simulink model "OutputMVA"  (Simulink 8.7)
settings: Solver=ode45  StartTime=0.0  StopTime=10.0  RelTol=1e-3
undefined symbols (not defined in the file or in its folder): sMP
(part 2 of 3)

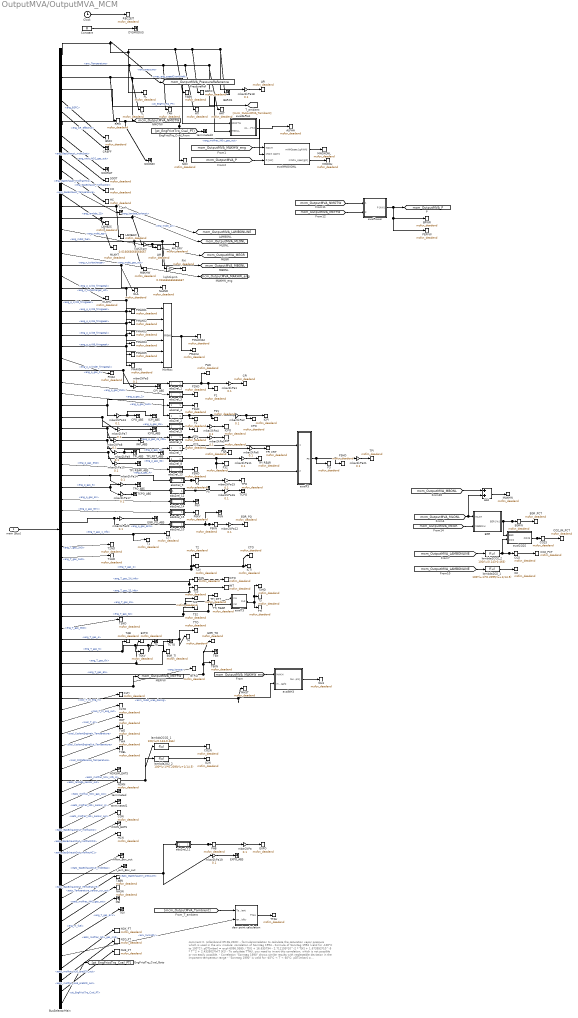
== system OutputMVA/OutputMVA_MCM ==
  note: comment C. Hillenbrand 09.06.2020:
      |
      | - formula/correlation to calculate the saturation vapor pressure which is used in the env module: correlation of Sonntag 1994
      | - Formula of Sonntag 1994 (valid for -100°C to 100°C): pDT[mbar] = exp(-6096.9385 / T[K] + 16.635794 - 2.711193*10^-2 * T[K] + 1.673952*10^-5 * T^2 + 2.433502*ln(T [K])
      | - To calculate TTAU, you need to invert this correlation, which is not possible or not easily possible.
      |
      | - Correlation "Sonntag 1990" shows similar results with neglectable deviation in the important temperatur range
      | - "Sonntag 1990" is valid for -45°C < T < 60°C:  pDT[mbar] = 6.112*exp((17.62*T)/(243.12+T))
      | - TTAU calculation:
      |                  h = pDT(TTAU) / pDT(T)
      |                  TTAU [°C] = 243.12 * ((17.62*T)/(243.12 + T) +ln(h))/((17.62*243.12)/(243.12 + T) -ln(h))   T=ambient temperatur    h=humidity
      |              (source: Beat P. Kneubuehl, "Ballistik: Theorie und Praxis" --> Kapitel 5.2.2 (Seite 155)
      |                           https://books.google.de/books?id=MtSBDwAAQBAJ&pg=PA155&lpg=PA155&dq=magnus+formel+s%C3%A4ttigungsdampfdruck+ballistik&source=bl&ots=gXIhdY-Apv&sig=ACfU3U0MpvOVRWRlQYtERQ3iZreJqlAHjg&hl=de&sa=X&ved=2ahUKEwic3uGe9fTpAhVzwcQBHcHJBsQQ6AEwAXoECAoQAQ#v=onepage&q=magnus%20formel%20s%C3%A4ttigungsdampfdruck%20ballistik&f=false
      |                      or: https://de.wikipedia.org/wiki/Sättigungsdampfdruck    --> Magnus-Formel)
      |
      |
      | --> The two correlations ("Sonntag 1994" and "Sonntag 1990" show results with negectable deviations in the important temperature range compared to MVAPC correlation.
      | --> Correlation "Sonntag 1994" will still be implemented in the environment modul.
      | --> For TTAU calculation "Sonntag 1990" will be used, due to the possible inversion the correlation.
  main [Bus] : Inport
  ALPHA : M-S-Function  Tag=VTOS_ALPHA  FunctionName=msfcn_deadend  mask(S-function: msfcn_deadend){}
      mask help: This is a level-2 M file S-function for communication with a VITOS (Virtual Testbench Operating System) display GUI element.
      mask Help: This is a level-2 M file S-function for communication with a VITOS (Virtual Testbench Operating System) display GUI element.
      mask Display: disp(['V'])
  AM : M-S-Function  Tag=VTOS_AM  FunctionName=msfcn_deadend  mask(S-function: msfcn_deadend){}
      mask help: This is a level-2 M file S-function for communication with a VITOS (Virtual Testbench Operating System) display GUI element.
      mask Help: This is a level-2 M file S-function for communication with a VITOS (Virtual Testbench Operating System) display GUI element.
      mask Display: disp(['V'])
  AMT : M-S-Function  Tag=VTOS_AMT  FunctionName=msfcn_deadend  mask(S-function: msfcn_deadend){}
      mask help: This is a level-2 M file S-function for communication with a VITOS (Virtual Testbench Operating System) display GUI element.
      mask Help: This is a level-2 M file S-function for communication with a VITOS (Virtual Testbench Operating System) display GUI element.
      mask Display: disp(['V'])
  AM_DRY : M-S-Function  Tag=VTOS_AM_DRY  FunctionName=msfcn_deadend  mask(S-function: msfcn_deadend){}
      mask help: This is a level-2 M file S-function for communication with a VITOS (Virtual Testbench Operating System) display GUI element.
      mask Help: This is a level-2 M file S-function for communication with a VITOS (Virtual Testbench Operating System) display GUI element.
      mask Display: disp(['V'])
  API : M-S-Function  Tag=VTOS_API  FunctionName=msfcn_deadend  mask(S-function: msfcn_deadend){}
      mask help: This is a level-2 M file S-function for communication with a VITOS (Virtual Testbench Operating System) display GUI element.
      mask Help: This is a level-2 M file S-function for communication with a VITOS (Virtual Testbench Operating System) display GUI element.
      mask Display: disp(['V'])
  ATI : M-S-Function  Tag=VTOS_ATI  FunctionName=msfcn_deadend  mask(S-function: msfcn_deadend){}
      mask help: This is a level-2 M file S-function for communication with a VITOS (Virtual Testbench Operating System) display GUI element.
      mask Help: This is a level-2 M file S-function for communication with a VITOS (Virtual Testbench Operating System) display GUI element.
      mask Display: disp(['V'])
  Add : Sum
  BARO : M-S-Function  Tag=VTOS_BARO  FunctionName=msfcn_deadend  mask(S-function: msfcn_deadend){}
      mask help: This is a level-2 M file S-function for communication with a VITOS (Virtual Testbench Operating System) display GUI element.
      mask Help: This is a level-2 M file S-function for communication with a VITOS (Virtual Testbench Operating System) display GUI element.
      mask Display: disp(['V'])
  BARO1 : Terminator
  BPWR : M-S-Function  Tag=VTOS_BPWR  FunctionName=msfcn_deadend  mask(S-function: msfcn_deadend){}
      mask help: This is a level-2 M file S-function for communication with a VITOS (Virtual Testbench Operating System) display GUI element.
      mask Help: This is a level-2 M file S-function for communication with a VITOS (Virtual Testbench Operating System) display GUI element.
      mask Display: disp(['V'])
  BSFC : M-S-Function  Tag=VTOS_BSFC  FunctionName=msfcn_deadend  mask(S-function: msfcn_deadend){}
      mask help: This is a level-2 M file S-function for communication with a VITOS (Virtual Testbench Operating System) display GUI element.
      mask Help: This is a level-2 M file S-function for communication with a VITOS (Virtual Testbench Operating System) display GUI element.
      mask Display: disp(['V'])
  BTRQ : M-S-Function  Tag=VTOS_BTRQ  FunctionName=msfcn_deadend  mask(S-function: msfcn_deadend){}
      mask help: This is a level-2 M file S-function for communication with a VITOS (Virtual Testbench Operating System) display GUI element.
      mask Help: This is a level-2 M file S-function for communication with a VITOS (Virtual Testbench Operating System) display GUI element.
      mask Display: disp(['V'])
  BusSelectorMain : BusSelector  OutputSignals=boundary [Bus].env_pressure,boundary [Bus].env_Temperature,sensor [Bus].mec_eng_speedCrankshaft,control [Bus].pt_EngTrq_Rq_PT,info [Bus].eng_BSFC,info [Bus].eng_CR_effective,sensor [Bus].eng_molfrac_NOx_gas_out,info [Bus].eng_ratio_NO2_gas_out,physics [Bus].eng_GasExhaust_mdotSoot,physics [Bus].eng_GasExhaust_molfracCO,physics [Bus].eng_GasExhaust_molfracHC1,physics [Bus].eng_GasExhaust_Temperature,info [Bus].eng_lambda_2S,sensor [Bus].eng_lambda_exhaust,sensor [Bus].eng_mdot_air,sensor [Bus].eng_mdot_egr,info [Bus].eng_mdot_fuel,sensor [Bus].eng_mdot_gas_out,sensor [Bus].eng_n_turbocharger,sensor [Bus].eng_n_turbocharger_HP,info [Bus].eng_p_cyl01_firingpeak,info [Bus].eng_p_cyl02_firingpeak,info [Bus].eng_p_cyl03_firingpeak,info [Bus].eng_p_cyl04_firingpeak,info [Bus].eng_p_cyl05_firingpeak,info [Bus].eng_p_cyl06_firingpeak,info [Bus].eng_p_cylinder_firingpeak,info [Bus].eng_p_gas_1,info [Bus].eng_p_gas_2ND,info [Bus].eng_p_gas_1HD,info [Bus].eng_p_gas_2,sensor [Bus].eng_p_gas_2N,info [Bus].eng_p_gas_2S_info,sensor [Bus].eng_p_gas_31,info [Bus].eng_p_gas_32,info [Bus].eng_p_gas_3ND,sensor [Bus].eng_p_gas_4,info [Bus].eng_p_gas_5,info [Bus].eng_p_gas_6V,info [Bus].eng_p_gas_6KV,sensor [Bus].eng_p_gas_6KN,info [Bus].eng_T_gas_1_info,info [Bus].eng_T_gas_2ND,info [Bus].eng_T_gas_1HD,sensor [Bus].eng_T_gas_2,info [Bus].eng_T_gas_2N_info,info [Bus].eng_T_gas_2S_info,sensor [Bus].eng_T_gas_31,sensor [Bus].eng_T_gas_32,info [Bus].eng_T_gas_3ND,sensor [Bus].eng_T_gas_4,info [Bus].eng_T_gas_5,info [Bus].eng_T_gas_6V,sensor [Bus].eng_T_gas_6N,sensor [Bus].eng_torque,actuator [Bus].acm_mdot_urea_dosing,sensor [Bus].cool_T_ct_eng_in,sensor [Bus].cool_T_ct_eng_out,sensor [Bus].cool_T_oil,physics [Bus].cool_CoolantEngineIn_Temperature,physics [Bus].cool_CoolantEngineOut_Temperature,physics [Bus].cool_OilReference_Temperature,sensor [Bus].eats_lambda_sensor_out,info [Bus].eats_molfrac_NOx_info_in,info [Bus].eats_molfrac_NOx_gas_out,sensor [Bus].eats_molfrac_NOx_sensor_in,sensor [Bus].eats_molfrac_NOx_sensor_out,physics [Bus].eats_GasExhaustOut_molfracCO,physics [Bus].eats_GasExhaustOut_molfracCO2,physics [Bus].eats_GasExhaustOut_molfracHC1,physics [Bus].eats_GasExhaustIn_pressure,physics [Bus].eats_GasExhaustOut_mdotGas,physics [Bus].eats_GasExhaustOut_Temperature,sensor [Bus].eats_Temperature_sensor_scr_out,info [Bus].eats_molfrac_NH3_gas_out,info [Bus].eng_m_fuel,info [Bus].eng_T_gas_6VV,boundary [Bus].env_humidity,info [Bus].eats_molfrac_NOx_gas_mid,info [Bus].eats_molfrac_N2O_preSCR_out,info [Bus].eats_molfrac_NH3_preSCR_out, control [Bus].pt_EngFrictTrq_Cval_PT
  CLTI : M-S-Function  Tag=VTOS_CLTI  FunctionName=msfcn_deadend  mask(S-function: msfcn_deadend){}
      mask help: This is a level-2 M file S-function for communication with a VITOS (Virtual Testbench Operating System) display GUI element.
      mask Help: This is a level-2 M file S-function for communication with a VITOS (Virtual Testbench Operating System) display GUI element.
      mask Display: disp(['V'])
  CLTO : M-S-Function  Tag=VTOS_CLTO  FunctionName=msfcn_deadend  mask(S-function: msfcn_deadend){}
      mask help: This is a level-2 M file S-function for communication with a VITOS (Virtual Testbench Operating System) display GUI element.
      mask Help: This is a level-2 M file S-function for communication with a VITOS (Virtual Testbench Operating System) display GUI element.
      mask Display: disp(['V'])
  CO : M-S-Function  Tag=VTOS_CO  FunctionName=msfcn_deadend  mask(S-function: msfcn_deadend){}
      mask help: This is a level-2 M file S-function for communication with a VITOS (Virtual Testbench Operating System) display GUI element.
      mask Help: This is a level-2 M file S-function for communication with a VITOS (Virtual Testbench Operating System) display GUI element.
      mask Display: disp(['V'])
  CO2 : M-S-Function  Tag=VTOS_CO2  FunctionName=msfcn_deadend  mask(S-function: msfcn_deadend){}
      mask help: This is a level-2 M file S-function for communication with a VITOS (Virtual Testbench Operating System) display GUI element.
      mask Help: This is a level-2 M file S-function for communication with a VITOS (Virtual Testbench Operating System) display GUI element.
      mask Display: disp(['V'])
  CO2N : M-S-Function  Tag=VTOS_CO2N  FunctionName=msfcn_deadend  mask(S-function: msfcn_deadend){}
      mask help: This is a level-2 M file S-function for communication with a VITOS (Virtual Testbench Operating System) display GUI element.
      mask Help: This is a level-2 M file S-function for communication with a VITOS (Virtual Testbench Operating System) display GUI element.
      mask Display: disp(['V'])
  CO2N_EATS : Terminator
  CO2S : M-S-Function  Tag=VTOS_CO2S  FunctionName=msfcn_deadend  mask(S-function: msfcn_deadend){}
      mask help: This is a level-2 M file S-function for communication with a VITOS (Virtual Testbench Operating System) display GUI element.
      mask Help: This is a level-2 M file S-function for communication with a VITOS (Virtual Testbench Operating System) display GUI element.
      mask Display: disp(['V'])
  CO2_IM_PCT : M-S-Function  Tag=VTOS_CO2_IM_PCT  FunctionName=msfcn_deadend  mask(S-function: msfcn_deadend){}
      mask help: This is a level-2 M file S-function for communication with a VITOS (Virtual Testbench Operating System) display GUI element.
      mask Help: This is a level-2 M file S-function for communication with a VITOS (Virtual Testbench Operating System) display GUI element.
      mask Display: disp(['V'])
  CO2_PCT : M-S-Function  Tag=VTOS_CO2_PCT  FunctionName=msfcn_deadend  mask(S-function: msfcn_deadend){}
      mask help: This is a level-2 M file S-function for communication with a VITOS (Virtual Testbench Operating System) display GUI element.
      mask Help: This is a level-2 M file S-function for communication with a VITOS (Virtual Testbench Operating System) display GUI element.
      mask Display: disp(['V'])
  CON : M-S-Function  Tag=VTOS_CON  FunctionName=msfcn_deadend  mask(S-function: msfcn_deadend){}
      mask help: This is a level-2 M file S-function for communication with a VITOS (Virtual Testbench Operating System) display GUI element.
      mask Help: This is a level-2 M file S-function for communication with a VITOS (Virtual Testbench Operating System) display GUI element.
      mask Display: disp(['V'])
  CPI : M-S-Function  Tag=VTOS_CPI  FunctionName=msfcn_deadend  mask(S-function: msfcn_deadend){}
      mask help: This is a level-2 M file S-function for communication with a VITOS (Virtual Testbench Operating System) display GUI element.
      mask Help: This is a level-2 M file S-function for communication with a VITOS (Virtual Testbench Operating System) display GUI element.
      mask Display: disp(['V'])
  CPI_ABS : Terminator
  CPO : M-S-Function  Tag=VTOS_CPO  FunctionName=msfcn_deadend  mask(S-function: msfcn_deadend){}
      mask help: This is a level-2 M file S-function for communication with a VITOS (Virtual Testbench Operating System) display GUI element.
      mask Help: This is a level-2 M file S-function for communication with a VITOS (Virtual Testbench Operating System) display GUI element.
      mask Display: disp(['V'])
  CPO_ABS : Terminator
  CREFF : Terminator
  CTI : M-S-Function  Tag=VTOS_CTI  FunctionName=msfcn_deadend  mask(S-function: msfcn_deadend){}
      mask help: This is a level-2 M file S-function for communication with a VITOS (Virtual Testbench Operating System) display GUI element.
      mask Help: This is a level-2 M file S-function for communication with a VITOS (Virtual Testbench Operating System) display GUI element.
      mask Display: disp(['V'])
  CTO : M-S-Function  Tag=VTOS_CTO  FunctionName=msfcn_deadend  mask(S-function: msfcn_deadend){}
      mask help: This is a level-2 M file S-function for communication with a VITOS (Virtual Testbench Operating System) display GUI element.
      mask Help: This is a level-2 M file S-function for communication with a VITOS (Virtual Testbench Operating System) display GUI element.
      mask Display: disp(['V'])
  Clock : Clock
  Constant : Constant  Value=8
  DYSMODUS : Terminator
  EGR : Subsystem
  EGRW : M-S-Function  Tag=VTOS_EGRW  FunctionName=msfcn_deadend  mask(S-function: msfcn_deadend){}
      mask help: This is a level-2 M file S-function for communication with a VITOS (Virtual Testbench Operating System) display GUI element.
      mask Help: This is a level-2 M file S-function for communication with a VITOS (Virtual Testbench Operating System) display GUI element.
      mask Display: disp(['V'])
  EGR_PCT : M-S-Function  Tag=VTOS_EGR_PCT  FunctionName=msfcn_deadend  mask(S-function: msfcn_deadend){}
      mask help: This is a level-2 M file S-function for communication with a VITOS (Virtual Testbench Operating System) display GUI element.
      mask Help: This is a level-2 M file S-function for communication with a VITOS (Virtual Testbench Operating System) display GUI element.
      mask Display: disp(['V'])
  EGR_PO : M-S-Function  Tag=VTOS_EGR_PO  FunctionName=msfcn_deadend  mask(S-function: msfcn_deadend){}
      mask help: This is a level-2 M file S-function for communication with a VITOS (Virtual Testbench Operating System) display GUI element.
      mask Help: This is a level-2 M file S-function for communication with a VITOS (Virtual Testbench Operating System) display GUI element.
      mask Display: disp(['V'])
  EGR_PO_ABS : Terminator
  EGR_TI : M-S-Function  Tag=VTOS_EGR_TI  FunctionName=msfcn_deadend  mask(S-function: msfcn_deadend){}
      mask help: This is a level-2 M file S-function for communication with a VITOS (Virtual Testbench Operating System) display GUI element.
      mask Help: This is a level-2 M file S-function for communication with a VITOS (Virtual Testbench Operating System) display GUI element.
      mask Display: disp(['V'])
  EGR_TO : M-S-Function  Tag=VTOS_EGR_TO  FunctionName=msfcn_deadend  mask(S-function: msfcn_deadend){}
      mask help: This is a level-2 M file S-function for communication with a VITOS (Virtual Testbench Operating System) display GUI element.
      mask Help: This is a level-2 M file S-function for communication with a VITOS (Virtual Testbench Operating System) display GUI element.
      mask Display: disp(['V'])
  EXPO : M-S-Function  Tag=VTOS_EXPO  FunctionName=msfcn_deadend  mask(S-function: msfcn_deadend){}
      mask help: This is a level-2 M file S-function for communication with a VITOS (Virtual Testbench Operating System) display GUI element.
      mask Help: This is a level-2 M file S-function for communication with a VITOS (Virtual Testbench Operating System) display GUI element.
      mask Display: disp(['V'])
  EXPO_ABS : Terminator
  EXTO : M-S-Function  Tag=VTOS_EXTO  FunctionName=msfcn_deadend  mask(S-function: msfcn_deadend){}
      mask help: This is a level-2 M file S-function for communication with a VITOS (Virtual Testbench Operating System) display GUI element.
      mask Help: This is a level-2 M file S-function for communication with a VITOS (Virtual Testbench Operating System) display GUI element.
      mask Display: disp(['V'])
  FM : M-S-Function  Tag=VTOS_FM  FunctionName=msfcn_deadend  mask(S-function: msfcn_deadend){}
      mask help: This is a level-2 M file S-function for communication with a VITOS (Virtual Testbench Operating System) display GUI element.
      mask Help: This is a level-2 M file S-function for communication with a VITOS (Virtual Testbench Operating System) display GUI element.
      mask Display: disp(['V'])
  GOT : M-S-Function  Tag=VTOS_GOT  FunctionName=msfcn_deadend  mask(S-function: msfcn_deadend){}
      mask help: This is a level-2 M file S-function for communication with a VITOS (Virtual Testbench Operating System) display GUI element.
      mask Help: This is a level-2 M file S-function for communication with a VITOS (Virtual Testbench Operating System) display GUI element.
      mask Display: disp(['V'])
  HC : M-S-Function  Tag=VTOS_HC  FunctionName=msfcn_deadend  mask(S-function: msfcn_deadend){}
      mask help: This is a level-2 M file S-function for communication with a VITOS (Virtual Testbench Operating System) display GUI element.
      mask Help: This is a level-2 M file S-function for communication with a VITOS (Virtual Testbench Operating System) display GUI element.
      mask Display: disp(['V'])
  HCN : M-S-Function  Tag=VTOS_HCN  FunctionName=msfcn_deadend  mask(S-function: msfcn_deadend){}
      mask help: This is a level-2 M file S-function for communication with a VITOS (Virtual Testbench Operating System) display GUI element.
      mask Help: This is a level-2 M file S-function for communication with a VITOS (Virtual Testbench Operating System) display GUI element.
      mask Display: disp(['V'])
  ICPI : M-S-Function  Tag=VTOS_ICPI  FunctionName=msfcn_deadend  mask(S-function: msfcn_deadend){}
      mask help: This is a level-2 M file S-function for communication with a VITOS (Virtual Testbench Operating System) display GUI element.
      mask Help: This is a level-2 M file S-function for communication with a VITOS (Virtual Testbench Operating System) display GUI element.
      mask Display: disp(['V'])
  ICPI_ABS : Terminator
  ICPO : M-S-Function  Tag=VTOS_ICPO  FunctionName=msfcn_deadend  mask(S-function: msfcn_deadend){}
      mask help: This is a level-2 M file S-function for communication with a VITOS (Virtual Testbench Operating System) display GUI element.
      mask Help: This is a level-2 M file S-function for communication with a VITOS (Virtual Testbench Operating System) display GUI element.
      mask Display: disp(['V'])
  ICPO_ABS : Terminator
  ICTI : M-S-Function  Tag=VTOS_ICTI  FunctionName=msfcn_deadend  mask(S-function: msfcn_deadend){}
      mask help: This is a level-2 M file S-function for communication with a VITOS (Virtual Testbench Operating System) display GUI element.
      mask Help: This is a level-2 M file S-function for communication with a VITOS (Virtual Testbench Operating System) display GUI element.
      mask Display: disp(['V'])
  ICTO : M-S-Function  Tag=VTOS_ICTO  FunctionName=msfcn_deadend  mask(S-function: msfcn_deadend){}
      mask help: This is a level-2 M file S-function for communication with a VITOS (Virtual Testbench Operating System) display GUI element.
      mask Help: This is a level-2 M file S-function for communication with a VITOS (Virtual Testbench Operating System) display GUI element.
      mask Display: disp(['V'])
  IMP : M-S-Function  Tag=VTOS_IMP  FunctionName=msfcn_deadend  mask(S-function: msfcn_deadend){}
      mask help: This is a level-2 M file S-function for communication with a VITOS (Virtual Testbench Operating System) display GUI element.
      mask Help: This is a level-2 M file S-function for communication with a VITOS (Virtual Testbench Operating System) display GUI element.
      mask Display: disp(['V'])
  IMP_ABS : Terminator
  IMT : M-S-Function  Tag=VTOS_IMT  FunctionName=msfcn_deadend  mask(S-function: msfcn_deadend){}
      mask help: This is a level-2 M file S-function for communication with a VITOS (Virtual Testbench Operating System) display GUI element.
      mask Help: This is a level-2 M file S-function for communication with a VITOS (Virtual Testbench Operating System) display GUI element.
      mask Display: disp(['V'])
  LAMB2S : M-S-Function  Tag=VTOS_LAMB2S  FunctionName=msfcn_deadend  mask(S-function: msfcn_deadend){}
      mask help: This is a level-2 M file S-function for communication with a VITOS (Virtual Testbench Operating System) display GUI element.
      mask Help: This is a level-2 M file S-function for communication with a VITOS (Virtual Testbench Operating System) display GUI element.
      mask Display: disp(['V'])
  LAMBAW : M-S-Function  Tag=VTOS_LAMBAW  FunctionName=msfcn_deadend  mask(S-function: msfcn_deadend){}
      mask help: This is a level-2 M file S-function for communication with a VITOS (Virtual Testbench Operating System) display GUI element.
      mask Help: This is a level-2 M file S-function for communication with a VITOS (Virtual Testbench Operating System) display GUI element.
      mask Display: disp(['V'])
  MAKHW : M-S-Function  Tag=VTOS_MAKHW  FunctionName=msfcn_deadend  mask(S-function: msfcn_deadend){}
      mask help: This is a level-2 M file S-function for communication with a VITOS (Virtual Testbench Operating System) display GUI element.
      mask Help: This is a level-2 M file S-function for communication with a VITOS (Virtual Testbench Operating System) display GUI element.
      mask Display: disp(['V'])
  MB : Terminator
  MBKHW : M-S-Function  Tag=VTOS_MBKHW  FunctionName=msfcn_deadend  mask(S-function: msfcn_deadend){}
      mask help: This is a level-2 M file S-function for communication with a VITOS (Virtual Testbench Operating System) display GUI element.
      mask Help: This is a level-2 M file S-function for communication with a VITOS (Virtual Testbench Operating System) display GUI element.
      mask Display: disp(['V'])
  MHST : M-S-Function  Tag=VTOS_MHST  FunctionName=msfcn_deadend  mask(S-function: msfcn_deadend){}
      mask help: This is a level-2 M file S-function for communication with a VITOS (Virtual Testbench Operating System) display GUI element.
      mask Help: This is a level-2 M file S-function for communication with a VITOS (Virtual Testbench Operating System) display GUI element.
      mask Display: disp(['V'])
  MLKHT : M-S-Function  Tag=VTOS_MLKHT  FunctionName=msfcn_deadend  mask(S-function: msfcn_deadend){}
      mask help: This is a level-2 M file S-function for communication with a VITOS (Virtual Testbench Operating System) display GUI element.
      mask Help: This is a level-2 M file S-function for communication with a VITOS (Virtual Testbench Operating System) display GUI element.
      mask Display: disp(['V'])
  MNOXH : M-S-Function  Tag=VTOS_MNOXH  FunctionName=msfcn_deadend  mask(S-function: msfcn_deadend){}
      mask help: This is a level-2 M file S-function for communication with a VITOS (Virtual Testbench Operating System) display GUI element.
      mask Help: This is a level-2 M file S-function for communication with a VITOS (Virtual Testbench Operating System) display GUI element.
      mask Display: disp(['V'])
  MNOXONL : M-S-Function  Tag=VTOS_MNOXONL  FunctionName=msfcn_deadend  mask(S-function: msfcn_deadend){}
      mask help: This is a level-2 M file S-function for communication with a VITOS (Virtual Testbench Operating System) display GUI element.
      mask Help: This is a level-2 M file S-function for communication with a VITOS (Virtual Testbench Operating System) display GUI element.
      mask Display: disp(['V'])
  MinMax : MinMax  Function=max  Inputs=6
  N2O_FT : M-S-Function  Tag=VTOS_N2O_FT  FunctionName=msfcn_deadend  mask(S-function: msfcn_deadend){}
      mask help: This is a level-2 M file S-function for communication with a VITOS (Virtual Testbench Operating System) display GUI element.
      mask Help: This is a level-2 M file S-function for communication with a VITOS (Virtual Testbench Operating System) display GUI element.
      mask Display: disp(['V'])
  NH3 : M-S-Function  Tag=VTOS_NH3  FunctionName=msfcn_deadend  mask(S-function: msfcn_deadend){}
      mask help: This is a level-2 M file S-function for communication with a VITOS (Virtual Testbench Operating System) display GUI element.
      mask Help: This is a level-2 M file S-function for communication with a VITOS (Virtual Testbench Operating System) display GUI element.
      mask Display: disp(['V'])
  NH3N : M-S-Function  Tag=VTOS_NH3N  FunctionName=msfcn_deadend  mask(S-function: msfcn_deadend){}
      mask help: This is a level-2 M file S-function for communication with a VITOS (Virtual Testbench Operating System) display GUI element.
      mask Help: This is a level-2 M file S-function for communication with a VITOS (Virtual Testbench Operating System) display GUI element.
      mask Display: disp(['V'])
  NH3_FT : M-S-Function  Tag=VTOS_NH3_FT  FunctionName=msfcn_deadend  mask(S-function: msfcn_deadend){}
      mask help: This is a level-2 M file S-function for communication with a VITOS (Virtual Testbench Operating System) display GUI element.
      mask Help: This is a level-2 M file S-function for communication with a VITOS (Virtual Testbench Operating System) display GUI element.
      mask Display: disp(['V'])
  NLA : M-S-Function  Tag=VTOS_NLA  FunctionName=msfcn_deadend  mask(S-function: msfcn_deadend){}
      mask help: This is a level-2 M file S-function for communication with a VITOS (Virtual Testbench Operating System) display GUI element.
      mask Help: This is a level-2 M file S-function for communication with a VITOS (Virtual Testbench Operating System) display GUI element.
      mask Display: disp(['V'])
  NLAHD : M-S-Function  Tag=VTOS_NLAHD  FunctionName=msfcn_deadend  mask(S-function: msfcn_deadend){}
      mask help: This is a level-2 M file S-function for communication with a VITOS (Virtual Testbench Operating System) display GUI element.
      mask Help: This is a level-2 M file S-function for communication with a VITOS (Virtual Testbench Operating System) display GUI element.
      mask Display: disp(['V'])
  NLAND : M-S-Function  Tag=VTOS_NLAND  FunctionName=msfcn_deadend  mask(S-function: msfcn_deadend){}
      mask help: This is a level-2 M file S-function for communication with a VITOS (Virtual Testbench Operating System) display GUI element.
      mask Help: This is a level-2 M file S-function for communication with a VITOS (Virtual Testbench Operating System) display GUI element.
      mask Display: disp(['V'])
  NO2RAT : Terminator
  NOX : M-S-Function  Tag=VTOS_NOX  FunctionName=msfcn_deadend  mask(S-function: msfcn_deadend){}
      mask help: This is a level-2 M file S-function for communication with a VITOS (Virtual Testbench Operating System) display GUI element.
      mask Help: This is a level-2 M file S-function for communication with a VITOS (Virtual Testbench Operating System) display GUI element.
      mask Display: disp(['V'])
  NOXN : M-S-Function  Tag=VTOS_NOXN  FunctionName=msfcn_deadend  mask(S-function: msfcn_deadend){}
      mask help: This is a level-2 M file S-function for communication with a VITOS (Virtual Testbench Operating System) display GUI element.
      mask Help: This is a level-2 M file S-function for communication with a VITOS (Virtual Testbench Operating System) display GUI element.
      mask Display: disp(['V'])
  NOXSIM : Terminator
  NOXSIM_EATS : Terminator
  NOX_FT : M-S-Function  Tag=VTOS_NOX_FT  FunctionName=msfcn_deadend  mask(S-function: msfcn_deadend){}
      mask help: This is a level-2 M file S-function for communication with a VITOS (Virtual Testbench Operating System) display GUI element.
      mask Help: This is a level-2 M file S-function for communication with a VITOS (Virtual Testbench Operating System) display GUI element.
      mask Display: disp(['V'])
  O2 : M-S-Function  Tag=VTOS_O2  FunctionName=msfcn_deadend  mask(S-function: msfcn_deadend){}
      mask help: This is a level-2 M file S-function for communication with a VITOS (Virtual Testbench Operating System) display GUI element.
      mask Help: This is a level-2 M file S-function for communication with a VITOS (Virtual Testbench Operating System) display GUI element.
      mask Display: disp(['V'])
  O2N : M-S-Function  Tag=VTOS_O2N  FunctionName=msfcn_deadend  mask(S-function: msfcn_deadend){}
      mask help: This is a level-2 M file S-function for communication with a VITOS (Virtual Testbench Operating System) display GUI element.
      mask Help: This is a level-2 M file S-function for communication with a VITOS (Virtual Testbench Operating System) display GUI element.
      mask Display: disp(['V'])
  P1 : M-S-Function  Tag=VTOS_P1  FunctionName=msfcn_deadend  mask(S-function: msfcn_deadend){}
      mask help: This is a level-2 M file S-function for communication with a VITOS (Virtual Testbench Operating System) display GUI element.
      mask Help: This is a level-2 M file S-function for communication with a VITOS (Virtual Testbench Operating System) display GUI element.
      mask Display: disp(['V'])
  P1HD : M-S-Function  Tag=VTOS_P1HD  FunctionName=msfcn_deadend  mask(S-function: msfcn_deadend){}
      mask help: This is a level-2 M file S-function for communication with a VITOS (Virtual Testbench Operating System) display GUI element.
      mask Help: This is a level-2 M file S-function for communication with a VITOS (Virtual Testbench Operating System) display GUI element.
      mask Display: disp(['V'])
  P2 : M-S-Function  Tag=VTOS_P2  FunctionName=msfcn_deadend  mask(S-function: msfcn_deadend){}
      mask help: This is a level-2 M file S-function for communication with a VITOS (Virtual Testbench Operating System) display GUI element.
      mask Help: This is a level-2 M file S-function for communication with a VITOS (Virtual Testbench Operating System) display GUI element.
      mask Display: disp(['V'])
  P2N : M-S-Function  Tag=VTOS_P2N  FunctionName=msfcn_deadend  mask(S-function: msfcn_deadend){}
      mask help: This is a level-2 M file S-function for communication with a VITOS (Virtual Testbench Operating System) display GUI element.
      mask Help: This is a level-2 M file S-function for communication with a VITOS (Virtual Testbench Operating System) display GUI element.
      mask Display: disp(['V'])
  P2ND : M-S-Function  Tag=VTOS_P2ND  FunctionName=msfcn_deadend  mask(S-function: msfcn_deadend){}
      mask help: This is a level-2 M file S-function for communication with a VITOS (Virtual Testbench Operating System) display GUI element.
      mask Help: This is a level-2 M file S-function for communication with a VITOS (Virtual Testbench Operating System) display GUI element.
      mask Display: disp(['V'])
  P2S : M-S-Function  Tag=VTOS_P2S  FunctionName=msfcn_deadend  mask(S-function: msfcn_deadend){}
      mask help: This is a level-2 M file S-function for communication with a VITOS (Virtual Testbench Operating System) display GUI element.
      mask Help: This is a level-2 M file S-function for communication with a VITOS (Virtual Testbench Operating System) display GUI element.
      mask Display: disp(['V'])
  P2V : M-S-Function  Tag=VTOS_P2V  FunctionName=msfcn_deadend  mask(S-function: msfcn_deadend){}
      mask help: This is a level-2 M file S-function for communication with a VITOS (Virtual Testbench Operating System) display GUI element.
      mask Help: This is a level-2 M file S-function for communication with a VITOS (Virtual Testbench Operating System) display GUI element.
      mask Display: disp(['V'])
  P3 : M-S-Function  Tag=VTOS_P3  FunctionName=msfcn_deadend  mask(S-function: msfcn_deadend){}
      mask help: This is a level-2 M file S-function for communication with a VITOS (Virtual Testbench Operating System) display GUI element.
      mask Help: This is a level-2 M file S-function for communication with a VITOS (Virtual Testbench Operating System) display GUI element.
      mask Display: disp(['V'])
  P31 : M-S-Function  Tag=VTOS_P31  FunctionName=msfcn_deadend  mask(S-function: msfcn_deadend){}
      mask help: This is a level-2 M file S-function for communication with a VITOS (Virtual Testbench Operating System) display GUI element.
      mask Help: This is a level-2 M file S-function for communication with a VITOS (Virtual Testbench Operating System) display GUI element.
      mask Display: disp(['V'])
  P32 : M-S-Function  Tag=VTOS_P32  FunctionName=msfcn_deadend  mask(S-function: msfcn_deadend){}
      mask help: This is a level-2 M file S-function for communication with a VITOS (Virtual Testbench Operating System) display GUI element.
      mask Help: This is a level-2 M file S-function for communication with a VITOS (Virtual Testbench Operating System) display GUI element.
      mask Display: disp(['V'])
  P3HD : M-S-Function  Tag=VTOS_P3HD  FunctionName=msfcn_deadend  mask(S-function: msfcn_deadend){}
      mask help: This is a level-2 M file S-function for communication with a VITOS (Virtual Testbench Operating System) display GUI element.
      mask Help: This is a level-2 M file S-function for communication with a VITOS (Virtual Testbench Operating System) display GUI element.
      mask Display: disp(['V'])
  P3ND : M-S-Function  Tag=VTOS_P3ND  FunctionName=msfcn_deadend  mask(S-function: msfcn_deadend){}
      mask help: This is a level-2 M file S-function for communication with a VITOS (Virtual Testbench Operating System) display GUI element.
      mask Help: This is a level-2 M file S-function for communication with a VITOS (Virtual Testbench Operating System) display GUI element.
      mask Display: disp(['V'])
  P4 : M-S-Function  Tag=VTOS_P4  FunctionName=msfcn_deadend  mask(S-function: msfcn_deadend){}
      mask help: This is a level-2 M file S-function for communication with a VITOS (Virtual Testbench Operating System) display GUI element.
      mask Help: This is a level-2 M file S-function for communication with a VITOS (Virtual Testbench Operating System) display GUI element.
      mask Display: disp(['V'])
  P5 : Terminator
  P6KN : M-S-Function  Tag=VTOS_P6KN  FunctionName=msfcn_deadend  mask(S-function: msfcn_deadend){}
      mask help: This is a level-2 M file S-function for communication with a VITOS (Virtual Testbench Operating System) display GUI element.
      mask Help: This is a level-2 M file S-function for communication with a VITOS (Virtual Testbench Operating System) display GUI element.
      mask Display: disp(['V'])
  P6KV : M-S-Function  Tag=VTOS_P6KV  FunctionName=msfcn_deadend  mask(S-function: msfcn_deadend){}
      mask help: This is a level-2 M file S-function for communication with a VITOS (Virtual Testbench Operating System) display GUI element.
      mask Help: This is a level-2 M file S-function for communication with a VITOS (Virtual Testbench Operating System) display GUI element.
      mask Display: disp(['V'])
  P6N : Terminator
  P6V : Terminator
  PAB : M-S-Function  Tag=VTOS_PAB  FunctionName=msfcn_deadend  mask(S-function: msfcn_deadend){}
      mask help: This is a level-2 M file S-function for communication with a VITOS (Virtual Testbench Operating System) display GUI element.
      mask Help: This is a level-2 M file S-function for communication with a VITOS (Virtual Testbench Operating System) display GUI element.
      mask Display: disp(['V'])
  PABN : M-S-Function  Tag=VTOS_PABN  FunctionName=msfcn_deadend  mask(S-function: msfcn_deadend){}
      mask help: This is a level-2 M file S-function for communication with a VITOS (Virtual Testbench Operating System) display GUI element.
      mask Help: This is a level-2 M file S-function for communication with a VITOS (Virtual Testbench Operating System) display GUI element.
      mask Display: disp(['V'])
  PAN : M-S-Function  Tag=VTOS_PAN  FunctionName=msfcn_deadend  mask(S-function: msfcn_deadend){}
      mask help: This is a level-2 M file S-function for communication with a VITOS (Virtual Testbench Operating System) display GUI element.
      mask Help: This is a level-2 M file S-function for communication with a VITOS (Virtual Testbench Operating System) display GUI element.
      mask Display: disp(['V'])
  PEFFW : M-S-Function  Tag=VTOS_PEFFW  FunctionName=msfcn_deadend  mask(S-function: msfcn_deadend){}
      mask help: This is a level-2 M file S-function for communication with a VITOS (Virtual Testbench Operating System) display GUI element.
      mask Help: This is a level-2 M file S-function for communication with a VITOS (Virtual Testbench Operating System) display GUI element.
      mask Display: disp(['V'])
  PL : M-S-Function  Tag=VTOS_PL  FunctionName=msfcn_deadend  mask(S-function: msfcn_deadend){}
      mask help: This is a level-2 M file S-function for communication with a VITOS (Virtual Testbench Operating System) display GUI element.
      mask Help: This is a level-2 M file S-function for communication with a VITOS (Virtual Testbench Operating System) display GUI element.
      mask Display: disp(['V'])
  PMAX : M-S-Function  Tag=VTOS_PMAX  FunctionName=msfcn_deadend  mask(S-function: msfcn_deadend){}
      mask help: This is a level-2 M file S-function for communication with a VITOS (Virtual Testbench Operating System) display GUI element.
      mask Help: This is a level-2 M file S-function for communication with a VITOS (Virtual Testbench Operating System) display GUI element.
      mask Display: disp(['V'])
  PMAX01 : M-S-Function  Tag=VTOS_PMAX01  FunctionName=msfcn_deadend  mask(S-function: msfcn_deadend){}
      mask help: This is a level-2 M file S-function for communication with a VITOS (Virtual Testbench Operating System) display GUI element.
      mask Help: This is a level-2 M file S-function for communication with a VITOS (Virtual Testbench Operating System) display GUI element.
      mask Display: disp(['V'])
  PMAX02 : M-S-Function  Tag=VTOS_PMAX02  FunctionName=msfcn_deadend  mask(S-function: msfcn_deadend){}
      mask help: This is a level-2 M file S-function for communication with a VITOS (Virtual Testbench Operating System) display GUI element.
      mask Help: This is a level-2 M file S-function for communication with a VITOS (Virtual Testbench Operating System) display GUI element.
      mask Display: disp(['V'])
  PMAX03 : M-S-Function  Tag=VTOS_PMAX03  FunctionName=msfcn_deadend  mask(S-function: msfcn_deadend){}
      mask help: This is a level-2 M file S-function for communication with a VITOS (Virtual Testbench Operating System) display GUI element.
      mask Help: This is a level-2 M file S-function for communication with a VITOS (Virtual Testbench Operating System) display GUI element.
      mask Display: disp(['V'])
  PMAX04 : M-S-Function  Tag=VTOS_PMAX04  FunctionName=msfcn_deadend  mask(S-function: msfcn_deadend){}
      mask help: This is a level-2 M file S-function for communication with a VITOS (Virtual Testbench Operating System) display GUI element.
      mask Help: This is a level-2 M file S-function for communication with a VITOS (Virtual Testbench Operating System) display GUI element.
      mask Display: disp(['V'])
  PMAX05 : M-S-Function  Tag=VTOS_PMAX05  FunctionName=msfcn_deadend  mask(S-function: msfcn_deadend){}
      mask help: This is a level-2 M file S-function for communication with a VITOS (Virtual Testbench Operating System) display GUI element.
      mask Help: This is a level-2 M file S-function for communication with a VITOS (Virtual Testbench Operating System) display GUI element.
      mask Display: disp(['V'])
  PMAX06 : M-S-Function  Tag=VTOS_PMAX06  FunctionName=msfcn_deadend  mask(S-function: msfcn_deadend){}
      mask help: This is a level-2 M file S-function for communication with a VITOS (Virtual Testbench Operating System) display GUI element.
      mask Help: This is a level-2 M file S-function for communication with a VITOS (Virtual Testbench Operating System) display GUI element.
      mask Display: disp(['V'])
  PMAXH : M-S-Function  Tag=VTOS_PMAXH  FunctionName=msfcn_deadend  mask(S-function: msfcn_deadend){}
      mask help: This is a level-2 M file S-function for communication with a VITOS (Virtual Testbench Operating System) display GUI element.
      mask Help: This is a level-2 M file S-function for communication with a VITOS (Virtual Testbench Operating System) display GUI element.
      mask Display: disp(['V'])
  PMAXMAX : M-S-Function  Tag=VTOS_PMAXMAX  FunctionName=msfcn_deadend  mask(S-function: msfcn_deadend){}
      mask help: This is a level-2 M file S-function for communication with a VITOS (Virtual Testbench Operating System) display GUI element.
      mask Help: This is a level-2 M file S-function for communication with a VITOS (Virtual Testbench Operating System) display GUI element.
      mask Display: disp(['V'])
  RECZEIT : M-S-Function  Tag=VTOS_RECZEIT  FunctionName=msfcn_deadend  mask(S-function: msfcn_deadend){}
      mask help: This is a level-2 M file S-function for communication with a VITOS (Virtual Testbench Operating System) display GUI element.
      mask Help: This is a level-2 M file S-function for communication with a VITOS (Virtual Testbench Operating System) display GUI element.
      mask Display: disp(['V'])
  RPM : M-S-Function  Tag=VTOS_RPM  FunctionName=msfcn_deadend  mask(S-function: msfcn_deadend){}
      mask help: This is a level-2 M file S-function for communication with a VITOS (Virtual Testbench Operating System) display GUI element.
      mask Help: This is a level-2 M file S-function for communication with a VITOS (Virtual Testbench Operating System) display GUI element.
      mask Display: disp(['V'])
  SOOT : M-S-Function  Tag=VTOS_SOOT  FunctionName=msfcn_deadend  mask(S-function: msfcn_deadend){}
      mask help: This is a level-2 M file S-function for communication with a VITOS (Virtual Testbench Operating System) display GUI element.
      mask Help: This is a level-2 M file S-function for communication with a VITOS (Virtual Testbench Operating System) display GUI element.
      mask Display: disp(['V'])
  T1 : M-S-Function  Tag=VTOS_T1  FunctionName=msfcn_deadend  mask(S-function: msfcn_deadend){}
      mask help: This is a level-2 M file S-function for communication with a VITOS (Virtual Testbench Operating System) display GUI element.
      mask Help: This is a level-2 M file S-function for communication with a VITOS (Virtual Testbench Operating System) display GUI element.
      mask Display: disp(['V'])
  T1HD : M-S-Function  Tag=VTOS_T1HD  FunctionName=msfcn_deadend  mask(S-function: msfcn_deadend){}
      mask help: This is a level-2 M file S-function for communication with a VITOS (Virtual Testbench Operating System) display GUI element.
      mask Help: This is a level-2 M file S-function for communication with a VITOS (Virtual Testbench Operating System) display GUI element.
      mask Display: disp(['V'])
  T2 : M-S-Function  Tag=VTOS_T2  FunctionName=msfcn_deadend  mask(S-function: msfcn_deadend){}
      mask help: This is a level-2 M file S-function for communication with a VITOS (Virtual Testbench Operating System) display GUI element.
      mask Help: This is a level-2 M file S-function for communication with a VITOS (Virtual Testbench Operating System) display GUI element.
      mask Display: disp(['V'])
  T2N : M-S-Function  Tag=VTOS_T2N  FunctionName=msfcn_deadend  mask(S-function: msfcn_deadend){}
      mask help: This is a level-2 M file S-function for communication with a VITOS (Virtual Testbench Operating System) display GUI element.
      mask Help: This is a level-2 M file S-function for communication with a VITOS (Virtual Testbench Operating System) display GUI element.
      mask Display: disp(['V'])
  T2ND : M-S-Function  Tag=VTOS_T2ND  FunctionName=msfcn_deadend  mask(S-function: msfcn_deadend){}
      mask help: This is a level-2 M file S-function for communication with a VITOS (Virtual Testbench Operating System) display GUI element.
      mask Help: This is a level-2 M file S-function for communication with a VITOS (Virtual Testbench Operating System) display GUI element.
      mask Display: disp(['V'])
  T2S : M-S-Function  Tag=VTOS_T2S  FunctionName=msfcn_deadend  mask(S-function: msfcn_deadend){}
      mask help: This is a level-2 M file S-function for communication with a VITOS (Virtual Testbench Operating System) display GUI element.
      mask Help: This is a level-2 M file S-function for communication with a VITOS (Virtual Testbench Operating System) display GUI element.
      mask Display: disp(['V'])
  T2V : M-S-Function  Tag=VTOS_T2V  FunctionName=msfcn_deadend  mask(S-function: msfcn_deadend){}
      mask help: This is a level-2 M file S-function for communication with a VITOS (Virtual Testbench Operating System) display GUI element.
      mask Help: This is a level-2 M file S-function for communication with a VITOS (Virtual Testbench Operating System) display GUI element.
      mask Display: disp(['V'])
  T3 : M-S-Function  Tag=VTOS_T3  FunctionName=msfcn_deadend  mask(S-function: msfcn_deadend){}
      mask help: This is a level-2 M file S-function for communication with a VITOS (Virtual Testbench Operating System) display GUI element.
      mask Help: This is a level-2 M file S-function for communication with a VITOS (Virtual Testbench Operating System) display GUI element.
      mask Display: disp(['V'])
  T31 : M-S-Function  Tag=VTOS_T31  FunctionName=msfcn_deadend  mask(S-function: msfcn_deadend){}
      mask help: This is a level-2 M file S-function for communication with a VITOS (Virtual Testbench Operating System) display GUI element.
      mask Help: This is a level-2 M file S-function for communication with a VITOS (Virtual Testbench Operating System) display GUI element.
      mask Display: disp(['V'])
  T32 : M-S-Function  Tag=VTOS_T32  FunctionName=msfcn_deadend  mask(S-function: msfcn_deadend){}
      mask help: This is a level-2 M file S-function for communication with a VITOS (Virtual Testbench Operating System) display GUI element.
      mask Help: This is a level-2 M file S-function for communication with a VITOS (Virtual Testbench Operating System) display GUI element.
      mask Display: disp(['V'])
  T3HD : M-S-Function  Tag=VTOS_T3HD  FunctionName=msfcn_deadend  mask(S-function: msfcn_deadend){}
      mask help: This is a level-2 M file S-function for communication with a VITOS (Virtual Testbench Operating System) display GUI element.
      mask Help: This is a level-2 M file S-function for communication with a VITOS (Virtual Testbench Operating System) display GUI element.
      mask Display: disp(['V'])
  T3ND : M-S-Function  Tag=VTOS_T3ND  FunctionName=msfcn_deadend  mask(S-function: msfcn_deadend){}
      mask help: This is a level-2 M file S-function for communication with a VITOS (Virtual Testbench Operating System) display GUI element.
      mask Help: This is a level-2 M file S-function for communication with a VITOS (Virtual Testbench Operating System) display GUI element.
      mask Display: disp(['V'])
  T4 : M-S-Function  Tag=VTOS_T4  FunctionName=msfcn_deadend  mask(S-function: msfcn_deadend){}
      mask help: This is a level-2 M file S-function for communication with a VITOS (Virtual Testbench Operating System) display GUI element.
      mask Help: This is a level-2 M file S-function for communication with a VITOS (Virtual Testbench Operating System) display GUI element.
      mask Display: disp(['V'])
  T5 : Terminator
  T6KN : M-S-Function  Tag=VTOS_T6KN  FunctionName=msfcn_deadend  mask(S-function: msfcn_deadend){}
      mask help: This is a level-2 M file S-function for communication with a VITOS (Virtual Testbench Operating System) display GUI element.
      mask Help: This is a level-2 M file S-function for communication with a VITOS (Virtual Testbench Operating System) display GUI element.
      mask Display: disp(['V'])
  T6KV : M-S-Function  Tag=VTOS_T6KV  FunctionName=msfcn_deadend  mask(S-function: msfcn_deadend){}
      mask help: This is a level-2 M file S-function for communication with a VITOS (Virtual Testbench Operating System) display GUI element.
      mask Help: This is a level-2 M file S-function for communication with a VITOS (Virtual Testbench Operating System) display GUI element.
      mask Display: disp(['V'])
  T6N : Terminator
  T6V : Terminator
  TAB : M-S-Function  Tag=VTOS_TAB  FunctionName=msfcn_deadend  mask(S-function: msfcn_deadend){}
      mask help: This is a level-2 M file S-function for communication with a VITOS (Virtual Testbench Operating System) display GUI element.
      mask Help: This is a level-2 M file S-function for communication with a VITOS (Virtual Testbench Operating System) display GUI element.
      mask Display: disp(['V'])
  TABN : M-S-Function  Tag=VTOS_TABN  FunctionName=msfcn_deadend  mask(S-function: msfcn_deadend){}
      mask help: This is a level-2 M file S-function for communication with a VITOS (Virtual Testbench Operating System) display GUI element.
      mask Help: This is a level-2 M file S-function for communication with a VITOS (Virtual Testbench Operating System) display GUI element.
      mask Display: disp(['V'])
  TAN : M-S-Function  Tag=VTOS_TAN  FunctionName=msfcn_deadend  mask(S-function: msfcn_deadend){}
      mask help: This is a level-2 M file S-function for communication with a VITOS (Virtual Testbench Operating System) display GUI element.
      mask Help: This is a level-2 M file S-function for communication with a VITOS (Virtual Testbench Operating System) display GUI element.
      mask Display: disp(['V'])
  TCPO : Terminator
  TCPO_ABS : Terminator
  TCTO : Terminator
  TL : M-S-Function  Tag=VTOS_TL  FunctionName=msfcn_deadend  mask(S-function: msfcn_deadend){}
      mask help: This is a level-2 M file S-function for communication with a VITOS (Virtual Testbench Operating System) display GUI element.
      mask Help: This is a level-2 M file S-function for communication with a VITOS (Virtual Testbench Operating System) display GUI element.
      mask Display: disp(['V'])
  TOEL : M-S-Function  Tag=VTOS_TOEL  FunctionName=msfcn_deadend  mask(S-function: msfcn_deadend){}
      mask help: This is a level-2 M file S-function for communication with a VITOS (Virtual Testbench Operating System) display GUI element.
      mask Help: This is a level-2 M file S-function for communication with a VITOS (Virtual Testbench Operating System) display GUI element.
      mask Display: disp(['V'])
  TPI : M-S-Function  Tag=VTOS_TPI  FunctionName=msfcn_deadend  mask(S-function: msfcn_deadend){}
      mask help: This is a level-2 M file S-function for communication with a VITOS (Virtual Testbench Operating System) display GUI element.
      mask Help: This is a level-2 M file S-function for communication with a VITOS (Virtual Testbench Operating System) display GUI element.
      mask Display: disp(['V'])
  TPI_ABS : Terminator
  TPI_FRT : M-S-Function  Tag=VTOS_TPI_FRT  FunctionName=msfcn_deadend  mask(S-function: msfcn_deadend){}
      mask help: This is a level-2 M file S-function for communication with a VITOS (Virtual Testbench Operating System) display GUI element.
      mask Help: This is a level-2 M file S-function for communication with a VITOS (Virtual Testbench Operating System) display GUI element.
      mask Display: disp(['V'])
  TPI_FRT_ABS : Terminator
  TPI_REAR : M-S-Function  Tag=VTOS_TPI_REAR  FunctionName=msfcn_deadend  mask(S-function: msfcn_deadend){}
      mask help: This is a level-2 M file S-function for communication with a VITOS (Virtual Testbench Operating System) display GUI element.
      mask Help: This is a level-2 M file S-function for communication with a VITOS (Virtual Testbench Operating System) display GUI element.
      mask Display: disp(['V'])
  TPI_REAR_ABS : Terminator
  TPO : M-S-Function  Tag=VTOS_TPO  FunctionName=msfcn_deadend  mask(S-function: msfcn_deadend){}
      mask help: This is a level-2 M file S-function for communication with a VITOS (Virtual Testbench Operating System) display GUI element.
      mask Help: This is a level-2 M file S-function for communication with a VITOS (Virtual Testbench Operating System) display GUI element.
      mask Display: disp(['V'])
  TPO_ABS : Terminator
  TTAU : M-S-Function  Tag=VTOS_TTAU  FunctionName=msfcn_deadend  mask(S-function: msfcn_deadend){}
      mask help: This is a level-2 M file S-function for communication with a VITOS (Virtual Testbench Operating System) display GUI element.
      mask Help: This is a level-2 M file S-function for communication with a VITOS (Virtual Testbench Operating System) display GUI element.
      mask Display: disp(['V'])
  TTI : M-S-Function  Tag=VTOS_TTI  FunctionName=msfcn_deadend  mask(S-function: msfcn_deadend){}
      mask help: This is a level-2 M file S-function for communication with a VITOS (Virtual Testbench Operating System) display GUI element.
      mask Help: This is a level-2 M file S-function for communication with a VITOS (Virtual Testbench Operating System) display GUI element.
      mask Display: disp(['V'])
  TTI_FRT : M-S-Function  Tag=VTOS_TTI_FRT  FunctionName=msfcn_deadend  mask(S-function: msfcn_deadend){}
      mask help: This is a level-2 M file S-function for communication with a VITOS (Virtual Testbench Operating System) display GUI element.
      mask Help: This is a level-2 M file S-function for communication with a VITOS (Virtual Testbench Operating System) display GUI element.
      mask Display: disp(['V'])
  TTI_REAR : M-S-Function  Tag=VTOS_TTI_REAR  FunctionName=msfcn_deadend  mask(S-function: msfcn_deadend){}
      mask help: This is a level-2 M file S-function for communication with a VITOS (Virtual Testbench Operating System) display GUI element.
      mask Help: This is a level-2 M file S-function for communication with a VITOS (Virtual Testbench Operating System) display GUI element.
      mask Display: disp(['V'])
  TTO : M-S-Function  Tag=VTOS_TTO  FunctionName=msfcn_deadend  mask(S-function: msfcn_deadend){}
      mask help: This is a level-2 M file S-function for communication with a VITOS (Virtual Testbench Operating System) display GUI element.
      mask Help: This is a level-2 M file S-function for communication with a VITOS (Virtual Testbench Operating System) display GUI element.
      mask Display: disp(['V'])
  TWA : M-S-Function  Tag=VTOS_TWA  FunctionName=msfcn_deadend  mask(S-function: msfcn_deadend){}
      mask help: This is a level-2 M file S-function for communication with a VITOS (Virtual Testbench Operating System) display GUI element.
      mask Help: This is a level-2 M file S-function for communication with a VITOS (Virtual Testbench Operating System) display GUI element.
      mask Display: disp(['V'])
  TWE : M-S-Function  Tag=VTOS_TWE  FunctionName=msfcn_deadend  mask(S-function: msfcn_deadend){}
      mask help: This is a level-2 M file S-function for communication with a VITOS (Virtual Testbench Operating System) display GUI element.
      mask Help: This is a level-2 M file S-function for communication with a VITOS (Virtual Testbench Operating System) display GUI element.
      mask Display: disp(['V'])
  T_exh : Terminator
  T_exh_Box_out : Terminator
  abs2rel_1 : Subsystem
  abs2rel_10 : Subsystem
  abs2rel_11 : Subsystem
  abs2rel_12 : Subsystem
  abs2rel_13 : Subsystem
  abs2rel_14 : Subsystem
  abs2rel_15 : Subsystem
  abs2rel_2 : Subsystem
  abs2rel_3 : Subsystem
  abs2rel_4 : Subsystem
  abs2rel_5 : Subsystem
  abs2rel_6 : Subsystem
  abs2rel_7 : Subsystem
  abs2rel_8 : Subsystem
  abs2rel_9 : Subsystem
  dew point calculation : Subsystem
  evalALPHA : Subsystem
  evalCO2S : Subsystem
  evalMNOXONL : Subsystem
  evalNH3 : Subsystem
  evalP3 : Subsystem
  evalPower : Subsystem
  evalT3 : Subsystem
  kgh2kgm : Gain  Gain=0.016666666666667
  kgh2kgm1 : Gain  Gain=0.016666666666667
  lambda2CO2_1 : Fcn  Expr=100/(u/0.143-0.466)
  lambda2CO2_2 : Fcn  Expr=100/(u/0.143-0.466)
  lambda2O2_1 : Fcn  Expr=100*(u-1)*0.2099/(u+1/14.5)
  lambda2O2_2 : Fcn  Expr=100*(u-1)*0.2099/(u+1/14.5)
  mbar2kPa{,1..21} (22 alike) : Gain  Gain=0.1
  mflow_Box_out : Terminator
  terminated : Terminator
  terminated1 : Terminator
  terminated2 : Terminator
  tag scope: mcm_OutputMVA_LAMBONLINE=global, mcm_OutputMVA_MAKHW_eng=global, mcm_OutputMVA_MBONL=global, mcm_OutputMVA_MEFFW=global, mcm_OutputMVA_MEGR=global, mcm_OutputMVA_MLONL=global, mcm_OutputMVA_NMOTW=global, mcm_OutputMVA_P=global, mcm_OutputMVA_PressureReference=global
  wires:
  Add/1 -> MAKHW/1
  mbar2kPa21/1 -> TPI/1
  evalP3/1(P3) -> P3/1, P3HD/1, mbar2kPa21/1
  abs2rel_15/1(pressure_relative) -> P6KV/1
  abs2rel_14/1(pressure_relative) -> P6V/1
  BusSelectorMain/40 -> abs2rel_15/1(pressure_absolute)  "<eng_p_gas_6KV>"
  BusSelectorMain/39 -> abs2rel_14/1(pressure_absolute)  "<eng_p_gas_6V>"
  abs2rel_13/1(pressure_relative) -> P3ND/1
  Clock/1 -> RECZEIT/1
  [mcm_OutputMVA_MEFFW] -> evalPower/2(M [Nm])
  [mcm_OutputMVA_NMOTW] -> evalPower/1(n [rpm])
  lambda2O2_1/1 -> O2/1
  [mcm_OutputMVA_LAMBONLINE] -> lambda2O2_1/1
  [mcm_OutputMVA_LAMBONLINE] -> lambda2CO2_2/1
  [mcm_OutputMVA_MLONL] -> Add/2, EGR/1(MLKH)
  [mcm_OutputMVA_MAKHW_eng] -> evalNH3/1(MAKH)
  evalNH3/1("NH3 [ppm] ") -> NH3/1
  BusSelectorMain/56 -> MHST/1, evalNH3/2(mHWL  [g/h])  "<acm_mdot_urea_dosing>"
  [mcm_OutputMVA_MBONL] -> Add/1
  evalPower/1(P [kW]) -> [mcm_OutputMVA_P], BPWR/1, PEFFW/1
  BusSelectorMain/3 -> RPM/1, evalALPHA/1(NMOTW), [mcm_OutputMVA_NMOTW]  "<mec_eng_speedCrankshaft>"
  Constant/1 -> DYSMODUS/1
  EGR/1("EGR [%] ") -> EGRW/1, EGR_PCT/1, evalCO2S/1(EGR)
  evalCO2S/1(CO2S) -> CO2S/1, CO2_IM_PCT/1
  lambda2CO2_2/1 -> evalCO2S/2(CO2), CO2/1, CO2_PCT/1
  BusSelectorMain/27 -> PMAX/1  "<eng_p_cylinder_firingpeak>"
  BusSelectorMain/37 -> abs2rel_9/1(pressure_absolute), mbar2kPa14/1  "<eng_p_gas_4>"
  abs2rel_10/1(pressure_relative) -> P6N/1, P6KN/1, mbar2kPa12/1
  abs2rel_9/1(pressure_relative) -> mbar2kPa15/1, P4/1
  abs2rel_8/1(pressure_relative) -> evalP3/2(P32), P32/1, mbar2kPa11/1
  abs2rel_7/1(pressure_relative) -> mbar2kPa6/1, P31/1, evalP3/1(P31)
  BusSelectorMain/33 -> abs2rel_6/1(pressure_absolute), mbar2kPa8/1  "<eng_p_gas_2S_info>"
  BusSelectorMain/32 -> mbar2kPa7/1, abs2rel_5/1(pressure_absolute)  "<eng_p_gas_2N>"
  BusSelectorMain/30 -> abs2rel_4/1(pressure_absolute)  "<eng_p_gas_1HD>"
  BusSelectorMain/29 -> abs2rel_3/1(pressure_absolute)  "<eng_p_gas_2ND>"
  abs2rel_6/1(pressure_relative) -> P2S/1, mbar2kPa5/1
  abs2rel_5/1(pressure_relative) -> P2N/1, mbar2kPa4/1
  abs2rel_4/1(pressure_relative) -> P1HD/1
  abs2rel_3/1(pressure_relative) -> P2ND/1
  abs2rel_2/1(pressure_relative) -> P2/1, mbar2kPa2/1, P2V/1
  abs2rel_1/1(pressure_relative) -> PAN/1, P1/1, mbar2kPa1/1
  BusSelectorMain/28 -> mbar2kPa3/1, abs2rel_1/1(pressure_absolute)  "<eng_p_gas_1>"
  BusSelectorMain/1 -> [mcm_OutputMVA_PressureReference], PL/1, BARO/1, BARO1/1, mbar2kPa18/1, PABN/1  "<env_pressure>"
  BusSelectorMain/2 -> TL/1, [mcm_OutputMVA_Tambient], AMT/1, ATI/1, TAN/1  "<env_Temperature>"
  BusSelectorMain/31 -> abs2rel_2/1(pressure_absolute), mbar2kPa13/1  "<eng_p_gas_2>"
  BusSelectorMain/38 -> mbar2kPa17/1, abs2rel_12/1(pressure_absolute)  "<eng_p_gas_5>"
  mbar2kPa1/1 -> CPI/1
  mbar2kPa2/1 -> CPO/1, ICPI/1
  mbar2kPa4/1 -> ICPO/1
  mbar2kPa5/1 -> IMP/1
  mbar2kPa6/1 -> TPI_FRT/1
  mbar2kPa3/1 -> CPI_ABS/1
  mbar2kPa7/1 -> ICPO_ABS/1
  mbar2kPa8/1 -> IMP_ABS/1
  mbar2kPa9/1 -> TPI_ABS/1, TPI_FRT_ABS/1
  mbar2kPa10/1 -> TPI_REAR_ABS/1
  mbar2kPa11/1 -> TPI_REAR/1
  mbar2kPa12/1 -> EGR_PO/1
  mbar2kPa13/1 -> ICPI_ABS/1, CPO_ABS/1
  abs2rel_12/1(pressure_relative) -> P5/1, mbar2kPa16/1
  mbar2kPa14/1 -> TPO_ABS/1
  mbar2kPa15/1 -> TPO/1
  mbar2kPa16/1 -> TCPO/1
  mbar2kPa17/1 -> TCPO_ABS/1
  mbar2kPa18/1 -> API/1
  mbar2kPa20/1 -> EGR_PO_ABS/1
  BusSelectorMain/65 -> NOXN/1  "<eats_molfrac_NOx_gas_out>"
  BusSelectorMain/6 -> CREFF/1  "<eng_CR_effective>"
  BusSelectorMain/5 -> BSFC/1  "<eng_BSFC>"
  BusSelectorMain/7 -> NOXSIM/1, evalMNOXONL/2(cNOX [ppm]), NOX/1  "<eng_molfrac_NOx_gas_out>"
  [mcm_OutputMVA_P] -> evalMNOXONL/3(P [kW])
  evalMNOXONL/1("mNH3spec [g/kWh] ") -> MNOXONL/1
  [mcm_OutputMVA_MAKHW_eng] -> evalMNOXONL/1(MAKH)
  BusSelectorMain/9 -> SOOT/1  "<eng_GasExhaust_mdotSoot>"
  BusSelectorMain/8 -> NO2RAT/1  "<eng_ratio_NO2_gas_out>"
  BusSelectorMain/11 -> HC/1  "<eng_GasExhaust_molfracHC1>"
  BusSelectorMain/10 -> CO/1  "<eng_GasExhaust_molfracCO>"
  BusSelectorMain/14 -> [mcm_OutputMVA_LAMBONLINE], LAMBAW/1  "<eng_lambda_exhaust>"
  BusSelectorMain/13 -> LAMB2S/1  "<eng_lambda_2S>"
  [mcm_OutputMVA_MEGR] -> EGR/2(MEGRKH)
  BusSelectorMain/20 -> NLAHD/1  "<eng_n_turbocharger_HP>"
  BusSelectorMain/19 -> NLAND/1, NLA/1  "<eng_n_turbocharger>"
  BusSelectorMain/18 -> [mcm_OutputMVA_MAKHW_eng]  "<eng_mdot_gas_out>"
  BusSelectorMain/15 -> MLKHT/1, kgh2kgm/1, [mcm_OutputMVA_MLONL]  "<eng_mdot_air>"
  BusSelectorMain/16 -> [mcm_OutputMVA_MEGR]  "<eng_mdot_egr>"
  kgh2kgm/1 -> AM_DRY/1, AM/1
  kgh2kgm1/1 -> FM/1
  BusSelectorMain/17 -> [mcm_OutputMVA_MBONL], kgh2kgm1/1, MBKHW/1  "<eng_mdot_fuel>"
  BusSelectorMain/21 -> PMAX01/1, MinMax/1  "<eng_p_cyl01_firingpeak>"
  BusSelectorMain/22 -> PMAX02/1, MinMax/2  "<eng_p_cyl02_firingpeak>"
  BusSelectorMain/23 -> PMAX03/1, MinMax/3  "<eng_p_cyl03_firingpeak>"
  BusSelectorMain/24 -> PMAX04/1, MinMax/4  "<eng_p_cyl04_firingpeak>"
  BusSelectorMain/25 -> MinMax/5, PMAX05/1  "<eng_p_cyl05_firingpeak>"
  BusSelectorMain/26 -> PMAX06/1, MinMax/6  "<eng_p_cyl06_firingpeak>"
  BusSelectorMain/34 -> mbar2kPa9/1, abs2rel_7/1(pressure_absolute)  "<eng_p_gas_31>"
  BusSelectorMain/35 -> mbar2kPa10/1, abs2rel_8/1(pressure_absolute)  "<eng_p_gas_32>"
  BusSelectorMain/36 -> abs2rel_13/1(pressure_absolute)  "<eng_p_gas_3ND>"
  BusSelectorMain/41 -> abs2rel_10/1(pressure_absolute), mbar2kPa20/1  "<eng_p_gas_6KN>"
  evalT3/1(Out) -> TTI/1, T3HD/1, T3/1
  BusSelectorMain/52 -> TCTO/1, T5/1, EXTO/1, TAB/1  "<eng_T_gas_5>"
  BusSelectorMain/54 -> T6N/1, EGR_TO/1, T6KN/1  "<eng_T_gas_6N>"
  BusSelectorMain/50 -> T3ND/1  "<eng_T_gas_3ND>"
  BusSelectorMain/49 -> evalT3/2(In2), TTI_REAR/1, T32/1  "<eng_T_gas_32>"
  BusSelectorMain/48 -> evalT3/1(In1), TTI_FRT/1, T31/1  "<eng_T_gas_31>"
  BusSelectorMain/47 -> T2S/1, IMT/1  "<eng_T_gas_2S_info>"
  BusSelectorMain/46 -> T2N/1, ICTO/1  "<eng_T_gas_2N_info>"
  BusSelectorMain/44 -> T1HD/1  "<eng_T_gas_1HD>"
  BusSelectorMain/43 -> T2ND/1  "<eng_T_gas_2ND>"
  BusSelectorMain/45 -> T2V/1, T2/1, CTO/1, ICTI/1  "<eng_T_gas_2>"
  BusSelectorMain/42 -> CTI/1, T1/1  "<eng_T_gas_1_info>"
  BusSelectorMain/53 -> EGR_TI/1, T6KV/1  "<eng_T_gas_6V>"
  BusSelectorMain/58 -> CLTO/1  "<cool_T_ct_eng_out>"
  BusSelectorMain/59 -> GOT/1  "<cool_T_oil>"
  BusSelectorMain/55 -> [mcm_OutputMVA_MEFFW], BTRQ/1  "<eng_torque>"
  BusSelectorMain/57 -> CLTI/1  "<cool_T_ct_eng_in>"
  BusSelectorMain/74 -> TABN/1  "<eats_Temperature_sensor_scr_out>"
  abs2rel_11/1(pressure_relative) -> mbar2kPa/1, PAB/1
  BusSelectorMain/71 -> mbar2kPa19/1, abs2rel_11/1(pressure_absolute)  "<eats_GasExhaustIn_pressure>"
  mbar2kPa/1 -> EXPO/1
  mbar2kPa19/1 -> EXPO_ABS/1
  BusSelectorMain/64 -> NOXSIM_EATS/1  "<eats_molfrac_NOx_info_in>"
  lambda2O2_2/1 -> O2N/1
  BusSelectorMain/63 -> lambda2CO2_1/1, lambda2O2_2/1  "<eats_lambda_sensor_out>"
  lambda2CO2_1/1 -> CO2N/1
  BusSelectorMain/68 -> CON/1  "<eats_GasExhaustOut_molfracCO>"
  BusSelectorMain/70 -> HCN/1  "<eats_GasExhaustOut_molfracHC1>"
  BusSelectorMain/67 -> terminated1/1  "<eats_molfrac_NOx_sensor_out>"
  BusSelectorMain/66 -> terminated/1  "<eats_molfrac_NOx_sensor_in>"
  BusSelectorMain/69 -> CO2N_EATS/1  "<eats_GasExhaustOut_molfracCO2>"
  BusSelectorMain/75 -> NH3N/1  "<eats_molfrac_NH3_gas_out>"
  BusSelectorMain/12 -> T_exh/1  "<eng_GasExhaust_Temperature>"
  BusSelectorMain/73 -> T_exh_Box_out/1  "<eats_GasExhaustOut_Temperature>"
  BusSelectorMain/72 -> mflow_Box_out/1  "<eats_GasExhaustOut_mdotGas>"
  BusSelectorMain/77 -> T6V/1  "<eng_T_gas_6VV>"
  main [Bus]/1 -> BusSelectorMain/1
  BusSelectorMain/51 -> TTO/1, T4/1  "<eng_T_gas_4>"
  BusSelectorMain/79 -> NOX_FT/1  "<eats_molfrac_NOx_gas_mid>"
  BusSelectorMain/80 -> N2O_FT/1  "<eats_molfrac_N2O_preSCR_out>"
  BusSelectorMain/81 -> NH3_FT/1  "<eats_molfrac_NH3_preSCR_out>"
  BusSelectorMain/60 -> TWE/1  "<cool_CoolantEngineIn_Temperature>"
  BusSelectorMain/61 -> TWA/1  "<cool_CoolantEngineOut_Temperature>"
  BusSelectorMain/62 -> TOEL/1  "<cool_OilReference_Temperature>"
  BusSelectorMain/82 -> [pt_EngFrictTrq_Cval_PT]  "<pt_EngFrictTrq_Cval_PT>"
  [mcm_OutputMVA_Tambient] -> dew point calculation/1(Tambient)
  BusSelectorMain/78 -> dew point calculation/2(env_humidity)  "<env_humidity>"
  dew point calculation/1(TTAU) -> TTAU/1
  BusSelectorMain/76 -> MB/1  "<eng_m_fuel>"
  evalMNOXONL/2(mNOx_spec[g/h]) -> MNOXH/1
  evalALPHA/1(ALPHA [%]) -> ALPHA/1
  BusSelectorMain/4 -> evalALPHA/2(MSOLL)  "<pt_EngTrq_Rq_PT>"
  [pt_EngFrictTrq_Cval_PT] -> terminated2/1
  MinMax/1 -> PMAXH/1, PMAXMAX/1
